simulink model "sim"  (R2024b)
settings: Solver=VariableStepAuto  StartTime=0.0  StopTime=20  RelTol=1e-3
values from neighbouring files (symbols this model uses):
  b = 2    [mFile.m]
  k = 3    [mFile.m]
  m1 = 2    [mFile.m]
settings Model: Creator=Ishak  LastModifiedBy=Ishak

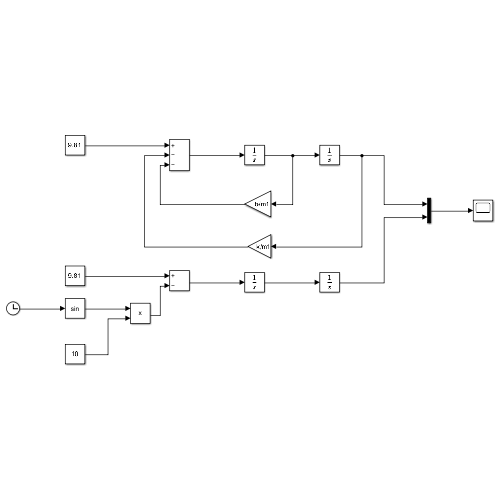
[thumbnail: Simulink's stored preview of the top-level diagram]
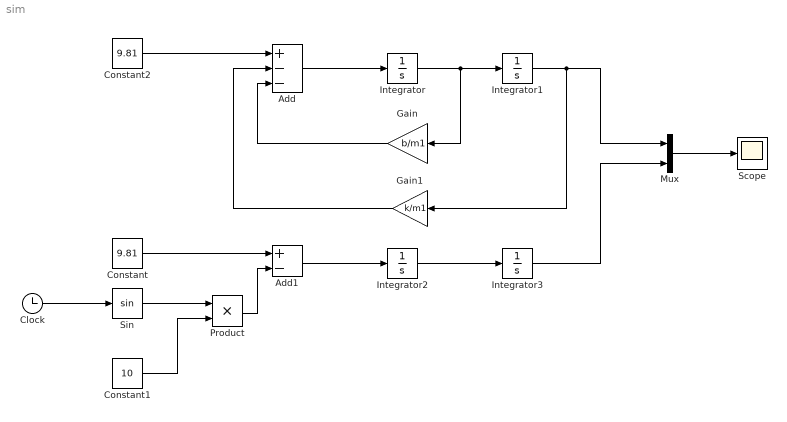
== system sim ==
  Add : Sum  Inputs=+--
  Add1 : Sum  Inputs=+-
  Clock : Clock
  Constant : Constant  Value=9.81
  Constant1 : Constant  Value=10
  Constant2 : Constant  Value=9.81
  Gain : Gain  Gain=b/m1
  Gain1 : Gain  Gain=k/m1
  Integrator{,1..3} (4 alike) : Integrator
  Mux : Mux  Inputs=2
  Product : Product
  Scope : Scope
  Sin : Trigonometry
  wires:
  Integrator/1 -> Gain/1, Integrator1/1
  Add/1 -> Integrator/1
  Integrator2/1 -> Integrator3/1
  Add1/1 -> Integrator2/1
  Constant/1 -> Add1/1
  Clock/1 -> Sin/1
  Product/1 -> Add1/2
  Constant1/1 -> Product/2
  Sin/1 -> Product/1
  Constant2/1 -> Add/1
  Integrator3/1 -> Mux/2
  Integrator1/1 -> Gain1/1, Mux/1
  Mux/1 -> Scope/1
  Gain/1 -> Add/3
  Gain1/1 -> Add/2
